simulink model "test_sf_bsearch"  (Simulink 7.7)
settings: Solver=FixedStepDiscrete  StartTime=0.0  StopTime=10.0  FixedStep=1  RelTol=1e-3
libraries: simulink x2
settings Model: Creator=lfeng  LastModifiedBy=lfeng

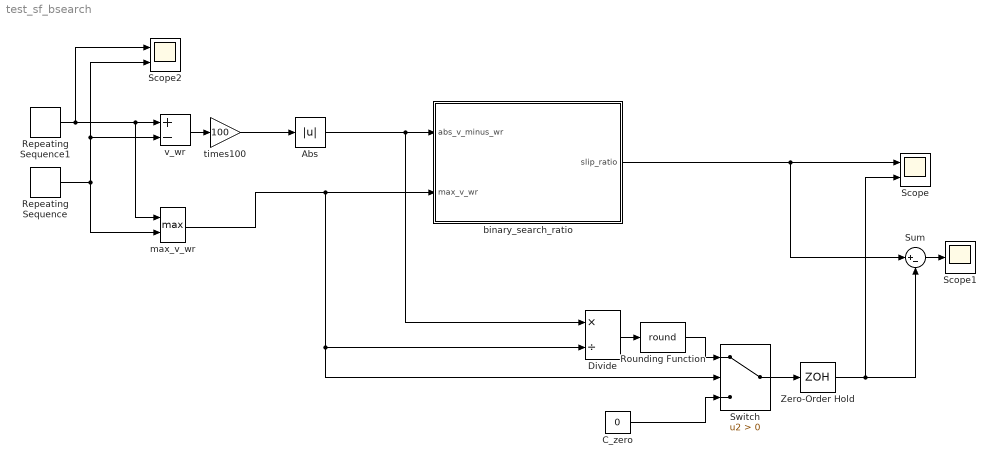
== system test_sf_bsearch ==
  Abs : Abs
  C_zero : Constant  Value=0
  Divide : Product  Inputs=*/
  Repeating Sequence : simulink/Sources/Repeating Sequence  SystemSampleTime=-1  rep_seq_t=[0 5 10]  rep_seq_y=[157 11 97]
  Repeating Sequence1 : simulink/Sources/Repeating Sequence  SystemSampleTime=-1  rep_seq_t=[0 4 8]  rep_seq_y=[0 99 0]
  Rounding Function : Rounding  Operator=round
  Scope : Scope  NumInputPorts=2
      settings: YMin=-5~-5  YMax=5~5
  Scope1 : Scope
  Scope2 : Scope  NumInputPorts=2
      settings: YMin=-5~-5  YMax=5~5  SaveName=ScopeData2
  Sum : Sum  Inputs=|+-
  Switch : Switch  Criteria=u2 > Threshold
  Zero-Order Hold : ZeroOrderHold
  binary_search_ratio : Stateflow chart  TreatAsAtomicUnit=on
  max_v_wr : MinMax  Function=max  Inputs=2
  times100 : Gain  Gain=100
  v_wr : Sum  Inputs=+-
  wires:
  binary_search_ratio/1(slip_ratio) -> Scope/1, Sum/1
  Divide/1 -> Rounding Function/1
  C_zero/1 -> Switch/3
  Switch/1 -> Zero-Order Hold/1
  Rounding Function/1 -> Switch/1
  max_v_wr/1 -> binary_search_ratio/2(max_v_wr), Divide/2, Switch/2
  v_wr/1 -> times100/1
  Repeating Sequence1/1 -> v_wr/1, max_v_wr/1, Scope2/1
  Repeating Sequence/1 -> max_v_wr/2, v_wr/2, Scope2/2
  times100/1 -> Abs/1
  Abs/1 -> binary_search_ratio/1(abs_v_minus_wr), Divide/1
  Zero-Order Hold/1 -> Scope/2, Sum/2
  Sum/1 -> Scope1/1

== stateflow chart binary_search_ratio ==
  (default) -> (junction 3) : /* check boundary conditions */
  (junction 3) -> (junction 5) [order 2]
  (junction 3) -> (junction 6) [order 1] : [abs_v_minus_wr == 0 || max_v_wr == 0]
  (junction 6) -> (junction 7) : {slip_ratio = 0;}
  (junction 5) -> (junction 8) [order 1] : [abs_v_minus_wr >= 100*max_v_wr]
  (junction 8) -> (junction 9) : {slip_ratio = 100;}
  (junction 5) -> (junction 11) [order 2] : {idx_min = 0;
      | idx_max = 99;} /* start binary search */
  (junction 11) -> (junction 10) [order 2] : [idx_max > idx_min]
  (junction 11) -> (junction 9) [order 3] : {slip_ratio = 20;}
      | /* if idx_max < idx_min, return 20%. The case should never happen */
  (junction 7) -> (junction 4) : /* terminate the flow */
  (junction 10) -> (junction 13) : {idx_mid = (idx_min + idx_max)/2;}
      | /* the middle index */
  (junction 13) -> (junction 14) [order 1] : [abs_v_minus_wr < idx_mid * max_v_wr]
      | /* if slip ratio is smaller than idx_mid */
  (junction 14) -> (junction 15) : {idx_max = idx_mid - 1;}
      | /* choose lower part */
  (junction 13) -> (junction 16) [order 2]
  (junction 16) -> (junction 17) [order 1] : [abs_v_minus_wr > (idx_mid + 1)*max_v_wr]
      | /* if slip ratio is larger than idx_mid + 1 */
  (junction 17) -> (junction 15) : {idx_min = idx_mid +1;}
      | /* choose upper part */
  (junction 16) -> (junction 18) [order 2]
  (junction 15) -> (junction 11) : /* go back for iterative search */
  (junction 18) -> (junction 19) [order 1] : [abs_v_minus_wr - idx_mid * max_v_wr <= (idx_mid + 1)*max_v_wr - abs_v_minus_wr]
      | /* if slip ratio is closer to idx_mid than idx_mid + 1 */
  (junction 19) -> (junction 4) : {slip_ratio = idx_mid;}
  (junction 18) -> (junction 12) [order 2] : {slip_ratio = idx_mid + 1;}
  (junction 4) -> (junction 12) : /* terminate the flow */
  (junction 9) -> (junction 7)
  (junction 11) -> (junction 20) [order 1] : [idx_max == idx_min]
      | /* decide if idx_min is idx_max
      | or idx_max + 1 */
  (junction 20) -> (junction 18) : {idx_mid = idx_max;}
  data: abs_v_minus_wr input double; max_v_wr input double; slip_ratio output double [0..100] =0; idx_mid local uint8 size=1 [0..99] =0; idx_min local uint8 size=1 [0..99] =0; idx_max local uint8 size=1 [0..99] =0
